simulink model "testNavigationSol"  (R2021a)
settings: Solver=VariableStepAuto  StartTime=0.0  StopTime=10.0  RelTol=1e-3
libraries: sharedtransform x1
settings Model: Creator=Laura  LastModifiedBy=Laura

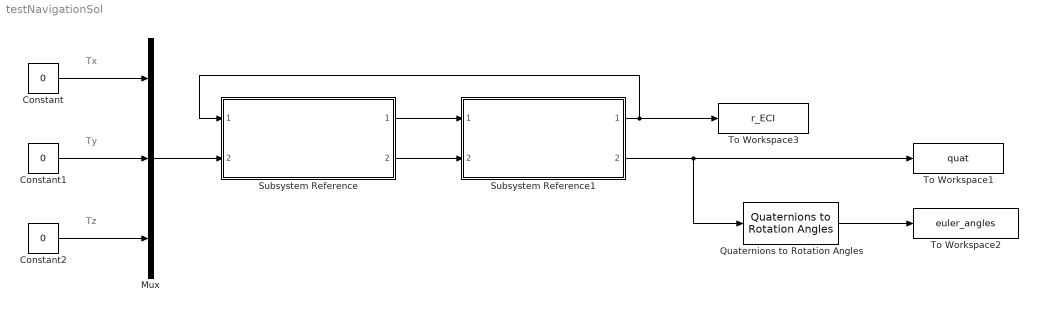
== system testNavigationSol ==
  note: Tz
  note: Ty
  note: Tx
  Constant : Constant  Value=0
  Constant1 : Constant  Value=0
  Constant2 : Constant  Value=0
  Mux : Mux  Inputs=3
  Quaternions to Rotation Angles : sharedtransform/Quaternions to Rotation Angles  rotationOrder=ZYX  aMode=aMode
      settings: SourceProductBaseCode=AE,PW,DR,MT,UV,VE
  Subsystem Reference : Subsystem  ReferencedSubsystem=Dynamics
  Subsystem Reference1 : Subsystem  ReferencedSubsystem=Kinematics
  To Workspace1 : ToWorkspace  VariableName=quat  SaveFormat=Timeseries  SampleTime=-1
  To Workspace2 : ToWorkspace  VariableName=euler_angles  SaveFormat=Timeseries  SampleTime=-1
  To Workspace3 : ToWorkspace  VariableName=r_ECI  SaveFormat=Timeseries  SampleTime=-1
  wires:
  Constant/1 -> Mux/1
  Constant1/1 -> Mux/2
  Subsystem Reference1/2 -> To Workspace1/1, Quaternions to Rotation Angles/1
  Subsystem Reference1/1 -> To Workspace3/1, Subsystem Reference/1
  Subsystem Reference/1 -> Subsystem Reference1/1
  Mux/1 -> Subsystem Reference/2
  Constant2/1 -> Mux/3
  Subsystem Reference/2 -> Subsystem Reference1/2
  Quaternions to Rotation Angles/1 -> To Workspace2/1
